simulink model "PD_model"  (R2022a)
settings: Solver=VariableStepAuto  StartTime=0.0  StopTime=10.0  RelTol=1e-3
settings Model: Creator=haowei  LastModifiedBy=haowei

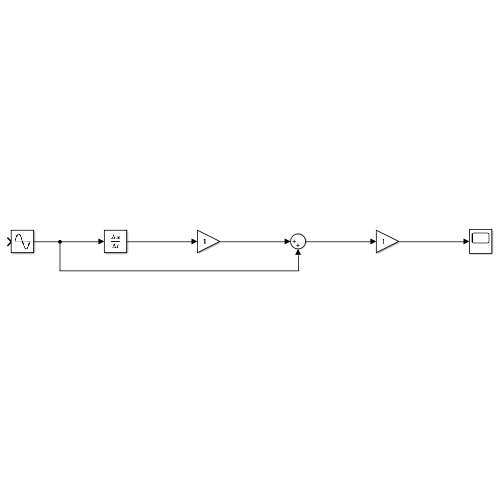
[thumbnail: Simulink's stored preview of the top-level diagram]
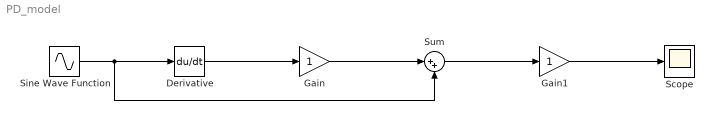
== system PD_model ==
  Derivative : Derivative
  Gain : Gain
  Gain1 : Gain
  Scope : Scope
  Sine Wave Function : Sin  TimeSource=Use external signal  SampleTime=0
  Sum : Sum  Inputs=|++
  wires:
  Derivative/1 -> Gain/1
  Gain/1 -> Sum/1
  Sum/1 -> Gain1/1
  Gain1/1 -> Scope/1
  Sine Wave Function/1 -> Sum/2, Derivative/1
